simulink model "UAVModel"  (R2018a)
settings: Solver=ode45  StartTime=0.0  StopTime=400  RelTol=1e-3  EnableMultiTasking=on
libraries: simulink x3, dspsrcs4 x1
settings Model: Creator=leo  LastModifiedBy=e357599
settings DataIOCC: LimitDataPoints=on  SaveFormat=Array  SignalLoggingSaveFormat=ModelDataLogs
settings OptimizationCC: ExpressionDepthLimit=2147483647  LifeSpan=inf
settings DebuggingCC: UnderspecifiedInitializationDetection=Classic  MergeDetectMultiDrivingBlocksExec=none  SolverPrmCheckMsg=warning  FcnCallInpInsideContextMsg=warning  StateNameClashWarn=warning  SFUnexpectedBacktrackingDiag=warning  SFNoUnconditionalDefaultTransitionDiag=warning  SFExecutionAtInitializationDiag=none
settings HardwareCC: ProdBitPerPointer=32  ProdBitPerSizeT=32  ProdBitPerPtrDiffT=32  ProdLargestAtomicFloat=None  ProdIntDivRoundTo=Undefined  ProdEndianess=Unspecified  ProdWordSize=32  ProdHWDeviceType=32-bit Generic
settings ModelReferenceCC: PropagateSignalLabelsOutOfModel=off
settings CodeAppCC: StateflowObjectComments=on
settings GRTTargetCC: TargetLangStandard=C89/C90 (ANSI)  GeneratePreprocessorConditionals=Disable all  CombineOutputUpdateFcns=off  GRTInterface=on
settings ConfigComp: CovMetricSettings=dw  CovHtmlReporting=on  CovSaveCumulativeToWorkspaceVar=on  CovSaveSingleToWorkspaceVar=on  CovExternalEMLEnable=off

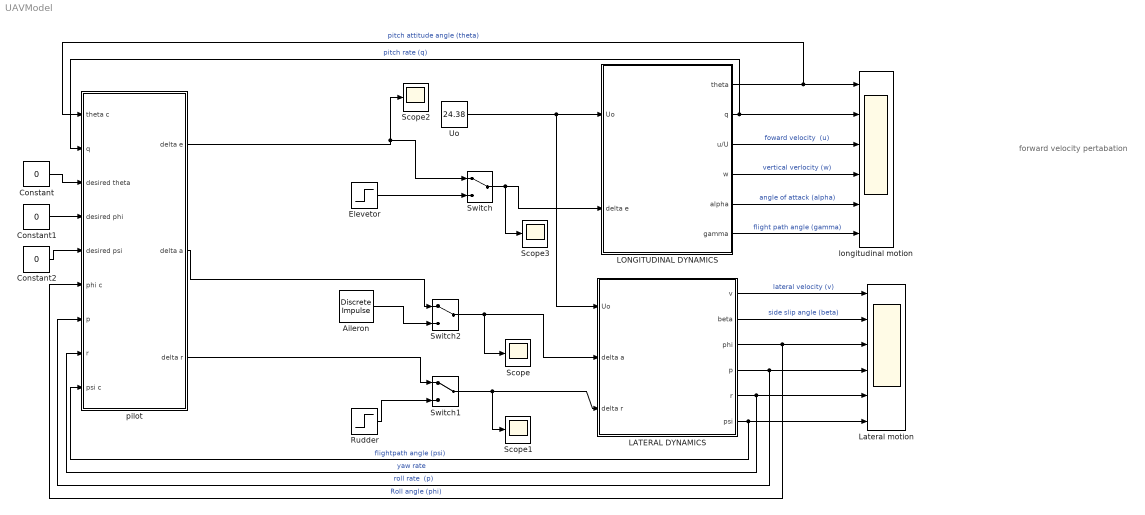
== system UAVModel ==
  note: forward velocity pertabation
  " Switch" : ManualSwitch
  " Switch1" : ManualSwitch
  " Switch2" : ManualSwitch
  Aileron : dspsrcs4/Discrete  Impulse  Delay=0  SampleTime=1  FrameSample=1  OutputFrames=off  dataType=double  isSigned=on  wordLen=16  udDataType=sfix(16)  fracBitsMode=Best precision  numFracBits=15  OutDataTypeStr=double  LastOutDataTypeStr=double
  Constant : Constant  Value=0  SampleTime=6
  Constant1 : Constant  Value=0
  Constant2 : Constant  Value=0
  Elevetor : Step  Time=0.5  After=-1  SampleTime=0
  LATERAL DYNAMICS : Subsystem
  LONGITUDINAL DYNAMICS : Subsystem
  Lateral motion : Scope  NumInputPorts=6
  Rudder : Step  Time=0.5  SampleTime=0
  Scope{,1..3} (4 alike) : Scope
  Uo : Constant  Value=24.38
  longitudinal motion : Scope  NumInputPorts=6
  "pilot " : Subsystem
  wires:
  " Switch"/1 -> Scope3/1, LONGITUDINAL DYNAMICS/2(delta e)
  Uo/1 -> LONGITUDINAL DYNAMICS/1(" Uo"), LATERAL DYNAMICS/1(Uo)
  Elevetor/1 -> " Switch"/2
  LONGITUDINAL DYNAMICS/6(gamma) -> longitudinal motion/6  "flight path angle (gamma)"
  " Switch1"/1 -> Scope1/1, LATERAL DYNAMICS/3(delta r)
  Rudder/1 -> " Switch1"/2
  LONGITUDINAL DYNAMICS/4(w) -> longitudinal motion/4  "vertical verlocity (w)"
  Constant1/1 -> "pilot "/4(desired phi)
  Constant2/1 -> "pilot "/5(desired psi)
  "pilot "/2(delta a) -> " Switch2"/1
  "pilot "/1(delta e) -> " Switch"/1, Scope2/1
  Constant/1 -> "pilot "/3(desired theta)
  "pilot "/3(delta r) -> " Switch1"/1
  LONGITUDINAL DYNAMICS/1(theta) -> longitudinal motion/1, "pilot "/1(theta c)  "pitch attitude angle (theta)"
  LONGITUDINAL DYNAMICS/2(q) -> longitudinal motion/2, "pilot "/2(q)  "pitch rate (q)"
  LONGITUDINAL DYNAMICS/3(u/U) -> longitudinal motion/3  "foward velocity  (u)"
  LONGITUDINAL DYNAMICS/5(alpha) -> longitudinal motion/5  "angle of attack (alpha)"
  LATERAL DYNAMICS/1(v) -> Lateral motion/1  "lateral velocity (v)"
  LATERAL DYNAMICS/2(beta) -> Lateral motion/2  "side slip angle (beta)"
  LATERAL DYNAMICS/3(phi) -> Lateral motion/3, "pilot "/6(phi c)  "Roll angle (phi)"
  LATERAL DYNAMICS/4(p) -> Lateral motion/4, "pilot "/7(p)  "roll rate  (p)"
  LATERAL DYNAMICS/5(r) -> Lateral motion/5, "pilot "/8(r)  "yaw rate"
  LATERAL DYNAMICS/6(psi) -> Lateral motion/6, "pilot "/9(psi c)  "flightpath angle (psi)"
  Aileron/1 -> " Switch2"/2
  " Switch2"/1 -> Scope/1, LATERAL DYNAMICS/2("delta a ")

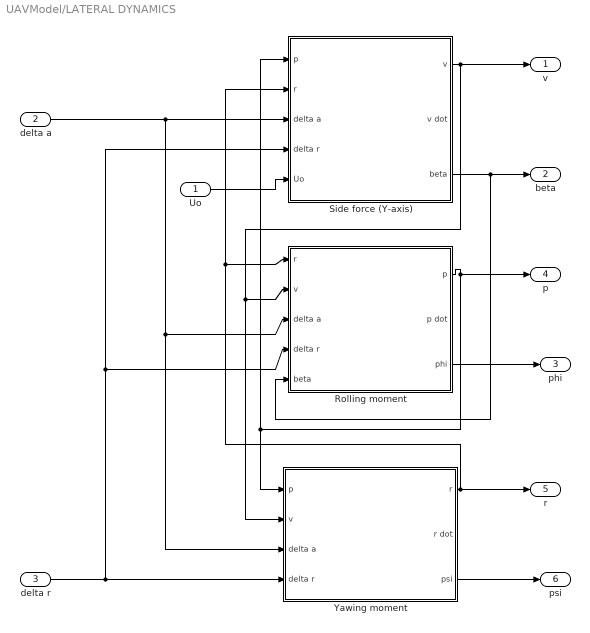
== system UAVModel/LATERAL DYNAMICS ==
  Uo : Inport
  "delta a " : Inport  Port=2
  delta r : Inport  Port=3
  Rolling moment : Subsystem
  Side force (Y-axis) : Subsystem
  Yawing moment : Subsystem
  v : Outport
  beta : Outport  Port=2
  phi : Outport  Port=3
  p : Outport  Port=4
  r : Outport  Port=5
  psi : Outport  Port=6
  wires:
  delta r/1 -> Side force (Y-axis)/4(delta r), Rolling moment/4(delta r), Yawing moment/4(delta r)
  "delta a "/1 -> Side force (Y-axis)/3(delta a), Rolling moment/3(delta a), Yawing moment/3(delta a)
  Uo/1 -> Side force (Y-axis)/5(Uo)
  Side force (Y-axis)/1(v) -> Rolling moment/2(v), Yawing moment/2(v), v/1
  Rolling moment/1(p) -> Yawing moment/1(p), Side force (Y-axis)/1(p), p/1
  Yawing moment/1(r) -> Rolling moment/1(r), Side force (Y-axis)/2(r), r/1
  Side force (Y-axis)/3(beta) -> beta/1, Rolling moment/5(beta)
  Yawing moment/3(psi) -> psi/1
  Rolling moment/3(phi) -> phi/1

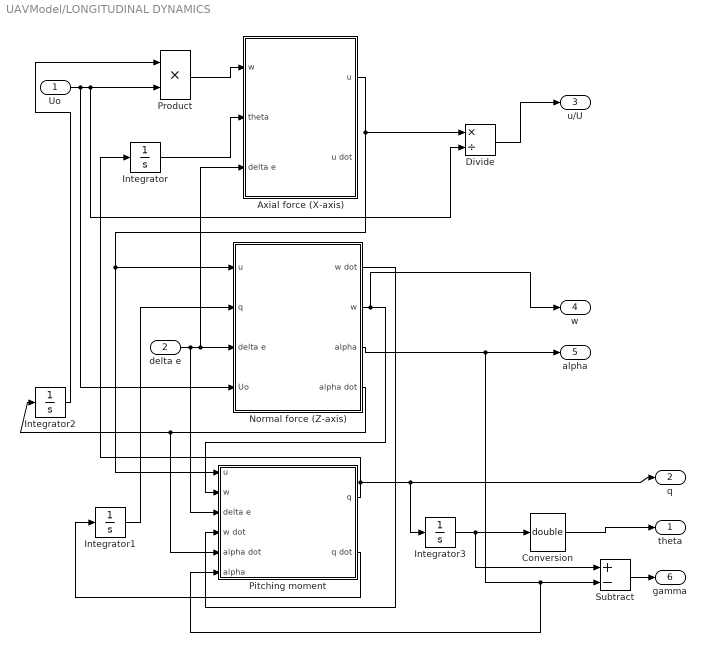
== system UAVModel/LONGITUDINAL DYNAMICS ==
  " Uo" : Inport
  delta e : Inport  Port=2
  " Conversion" : DataTypeConversion  OutDataTypeStr=double
  Axial force (X-axis) : Subsystem
  Divide : Product  Inputs=*/
  Integrator{,1..3} (4 alike) : Integrator
  "Normal force (Z-axis) " : Subsystem
  Pitching moment : Subsystem
  Product : Product  RndMeth=Zero
  Subtract : Sum  Inputs=+-
  theta : Outport
  q : Outport  Port=2
  u/U : Outport  Port=3
  w : Outport  Port=4
  alpha : Outport  Port=5
  gamma : Outport  Port=6
  wires:
  " Uo"/1 -> "Normal force (Z-axis) "/4(Uo), Product/2, Divide/2
  delta e/1 -> Pitching moment/3(delta e), "Normal force (Z-axis) "/3(delta e), Axial force (X-axis)/3(delta e)
  Product/1 -> Axial force (X-axis)/1(w)
  Axial force (X-axis)/1(u) -> Pitching moment/1(u), "Normal force (Z-axis) "/1(u), Divide/1
  "Normal force (Z-axis) "/2(w) -> Pitching moment/2(w), w/1
  "Normal force (Z-axis) "/1(w dot) -> Pitching moment/4(w dot)
  Pitching moment/1(q) -> Integrator/1, q/1, Integrator3/1
  Integrator/1 -> Axial force (X-axis)/2(theta)
  Integrator1/1 -> "Normal force (Z-axis) "/2(q)
  Pitching moment/2(q dot) -> Integrator1/1
  "Normal force (Z-axis) "/3(alpha) -> alpha/1, Subtract/2, Pitching moment/6("alpha ")
  Integrator2/1 -> Product/1
  "Normal force (Z-axis) "/4(alpha dot) -> Integrator2/1, Pitching moment/5(alpha dot)
  Integrator3/1 -> Subtract/1, " Conversion"/1
  Subtract/1 -> gamma/1
  " Conversion"/1 -> theta/1
  Divide/1 -> u/U/1

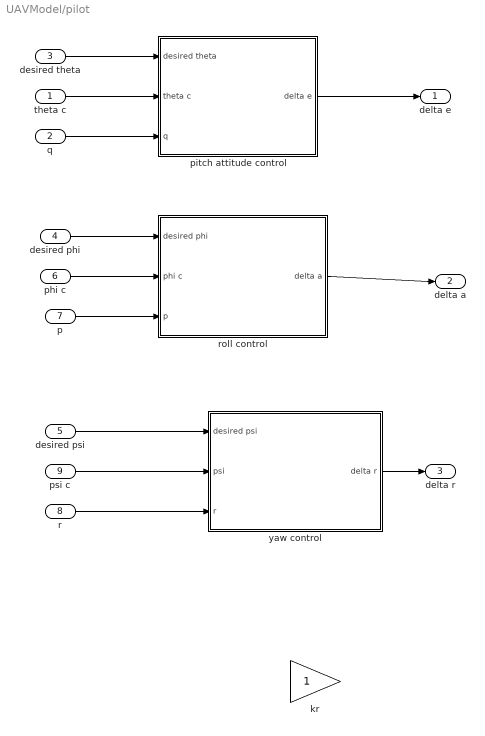
== system UAVModel/pilot  ==
  theta c : Inport
  q : Inport  Port=2
  desired theta : Inport  Port=3
  desired phi : Inport  Port=4
  desired psi : Inport  Port=5
  phi c : Inport  Port=6
  p : Inport  Port=7
  r : Inport  Port=8
  psi c : Inport  Port=9
  kr : Gain
  pitch attitude control : Subsystem
  roll control : Subsystem
  yaw control : Subsystem
  delta e : Outport
  delta a : Outport  Port=2
  delta r : Outport  Port=3
  wires:
  desired theta/1 -> pitch attitude control/1(desired theta)
  theta c/1 -> pitch attitude control/2(theta c)
  q/1 -> pitch attitude control/3(q)
  desired phi/1 -> roll control/1("desired phi ")
  phi c/1 -> roll control/2(phi c)
  p/1 -> roll control/3(p)
  desired psi/1 -> yaw control/1("desired psi ")
  psi c/1 -> yaw control/2(psi)
  r/1 -> yaw control/3(r)
  roll control/1(delta a) -> delta a/1
  pitch attitude control/1(delta e) -> delta e/1
  yaw control/1(delta r) -> delta r/1

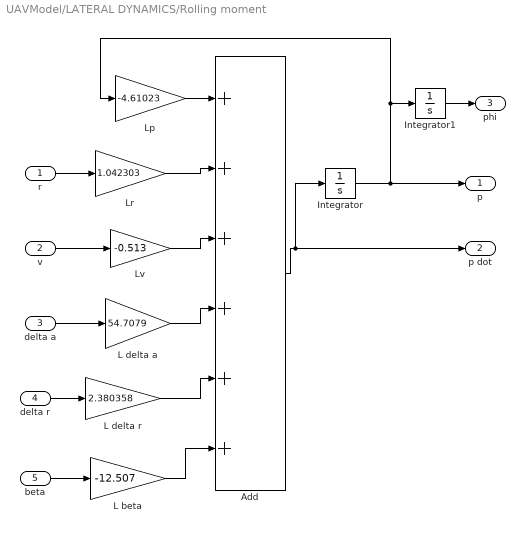
== system UAVModel/LATERAL DYNAMICS/Rolling moment ==
  r : Inport
  v : Inport  Port=2
  delta a : Inport  Port=3
  delta r : Inport  Port=4
  beta : Inport  Port=5
  Add : Sum  Inputs=++++++
  Integrator : Integrator
  Integrator1 : Integrator
  L beta : Gain  Gain=-12.507
  "L delta a " : Gain  Gain=54.7079
  L delta r : Gain  Gain=2.380358
  Lp : Gain  Gain=-4.61023
  Lr : Gain  Gain=1.042303
  Lv : Gain  Gain=-0.513
  p : Outport
  p dot : Outport  Port=2
  phi : Outport  Port=3
  wires:
  Add/1 -> p dot/1, Integrator/1
  Lp/1 -> Add/1
  Lr/1 -> Add/2
  Lv/1 -> Add/3
  "L delta a "/1 -> Add/4
  L delta r/1 -> Add/5
  delta r/1 -> L delta r/1
  delta a/1 -> "L delta a "/1
  v/1 -> Lv/1
  r/1 -> Lr/1
  Integrator/1 -> p/1, Lp/1, Integrator1/1
  Integrator1/1 -> phi/1
  L beta/1 -> Add/6
  beta/1 -> L beta/1

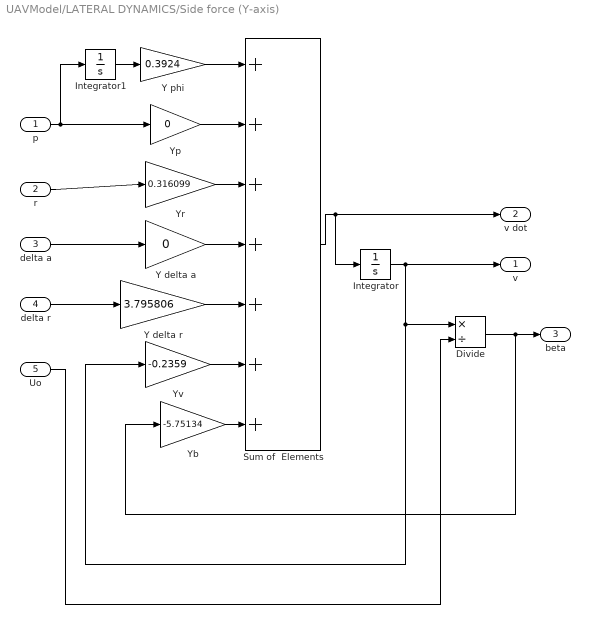
== system UAVModel/LATERAL DYNAMICS/Side force (Y-axis) ==
  p : Inport
  r : Inport  Port=2
  delta a : Inport  Port=3
  delta r : Inport  Port=4
  Uo : Inport  Port=5
  Divide : Product  Inputs=*/
  Integrator : Integrator
  Integrator1 : Integrator
  Sum of  Elements : Sum  Inputs=+++++++
  Y delta a : Gain  Gain=0
  Y delta r : Gain  Gain=3.795806
  Y phi : Gain  Gain=0.3924
  Yb : Gain  Gain=-5.75134
  Yp : Gain  Gain=0
  Yr : Gain  Gain=0.316099
  Yv : Gain  Gain=-0.2359
  v : Outport
  v dot : Outport  Port=2
  beta : Outport  Port=3
  wires:
  Sum of  Elements/1 -> v dot/1, Integrator/1
  Integrator/1 -> v/1, Divide/1, Yv/1
  Yv/1 -> Sum of  Elements/6
  Y delta r/1 -> Sum of  Elements/5
  Y delta a/1 -> Sum of  Elements/4
  Yr/1 -> Sum of  Elements/3
  Yp/1 -> Sum of  Elements/2
  Y phi/1 -> Sum of  Elements/1
  r/1 -> Yr/1
  p/1 -> Yp/1, Integrator1/1
  Integrator1/1 -> Y phi/1
  delta a/1 -> Y delta a/1
  delta r/1 -> Y delta r/1
  Uo/1 -> Divide/2
  Divide/1 -> beta/1, Yb/1
  Yb/1 -> Sum of  Elements/7

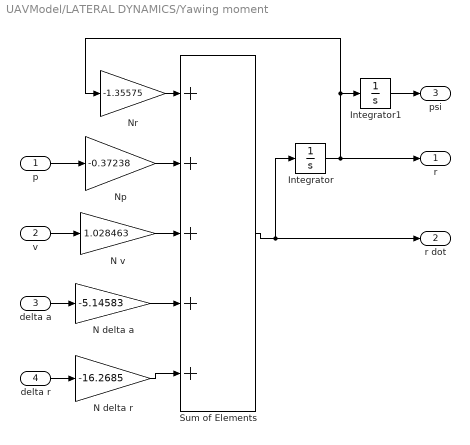
== system UAVModel/LATERAL DYNAMICS/Yawing moment ==
  p : Inport
  v : Inport  Port=2
  delta a : Inport  Port=3
  delta r : Inport  Port=4
  Integrator : Integrator
  Integrator1 : Integrator
  N delta a : Gain  Gain=-5.14583
  N delta r : Gain  Gain=-16.2685
  N v : Gain  Gain=1.028463
  Np : Gain  Gain=-0.37238
  Nr : Gain  Gain=-1.35575
  Sum of Elements : Sum  Inputs=+++++
  r : Outport
  r dot : Outport  Port=2
  psi : Outport  Port=3
  wires:
  Sum of Elements/1 -> Integrator/1, r dot/1
  Integrator/1 -> r/1, Nr/1, Integrator1/1
  delta r/1 -> N delta r/1
  delta a/1 -> N delta a/1
  v/1 -> N v/1
  p/1 -> Np/1
  Nr/1 -> Sum of Elements/1
  Np/1 -> Sum of Elements/2
  N v/1 -> Sum of Elements/3
  N delta a/1 -> Sum of Elements/4
  N delta r/1 -> Sum of Elements/5
  Integrator1/1 -> psi/1

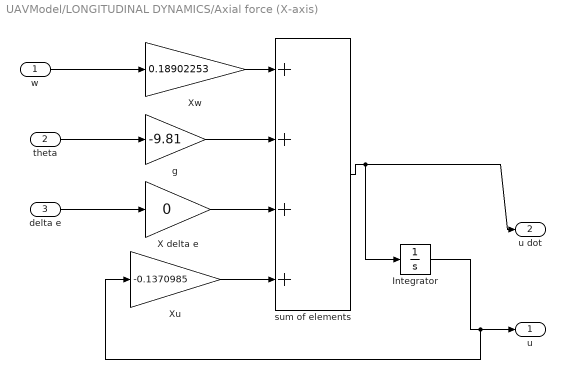
== system UAVModel/LONGITUDINAL DYNAMICS/Axial force (X-axis) ==
  w : Inport
  theta : Inport  Port=2
  delta e : Inport  Port=3
  Integrator : Integrator
  X delta e : Gain  Gain=0
  Xu : Gain  RequirementInfo={} %GIDa_afb63dbf_c4f0_45b2_8257_9555063e987b  Gain=-0.1370985
  Xw : Gain  Gain=0.18902253
  g : Gain  Gain=-9.81
  sum of elements : Sum  Inputs=++++
  u : Outport
  u dot : Outport  Port=2
  wires:
  Xw/1 -> sum of elements/1
  w/1 -> Xw/1
  g/1 -> sum of elements/2
  sum of elements/1 -> Integrator/1, u dot/1
  Integrator/1 -> Xu/1, u/1
  theta/1 -> g/1
  Xu/1 -> sum of elements/4
  X delta e/1 -> sum of elements/3
  delta e/1 -> X delta e/1

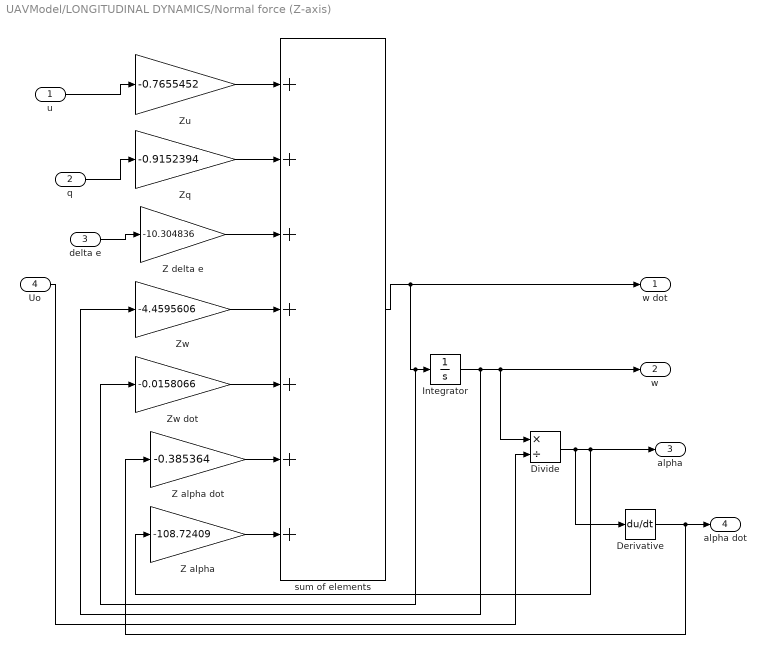
== system UAVModel/LONGITUDINAL DYNAMICS/Normal force (Z-axis)  ==
  u : Inport
  q : Inport  Port=2
  delta e : Inport  Port=3
  Uo : Inport  Port=4
  Derivative : Derivative
  Divide : Product  Inputs=*/
  Integrator : Integrator
  Z alpha : Gain  Gain=-108.72409
  Z alpha dot : Gain  Gain=-0.385364
  Z delta e : Gain  Gain=-10.304836
  Zq : Gain  Gain=-0.9152394
  Zu : Gain  Gain=-0.7655452
  Zw : Gain  Gain=-4.4595606
  Zw dot : Gain  Gain=-0.0158066
  sum of elements : Sum  Inputs=+++++++
  w dot : Outport
  w : Outport  Port=2
  alpha : Outport  Port=3
  alpha dot : Outport  Port=4
  wires:
  Zu/1 -> sum of elements/1
  u/1 -> Zu/1
  Zq/1 -> sum of elements/2
  q/1 -> Zq/1
  Z delta e/1 -> sum of elements/3
  delta e/1 -> Z delta e/1
  Zw/1 -> sum of elements/4
  sum of elements/1 -> w dot/1, Integrator/1, Zw dot/1
  Integrator/1 -> w/1, Divide/1, Zw/1
  Uo/1 -> Divide/2
  Divide/1 -> Derivative/1, alpha/1, Z alpha/1
  Derivative/1 -> alpha dot/1, Z alpha dot/1
  Zw dot/1 -> sum of elements/5
  Z alpha dot/1 -> sum of elements/6
  Z alpha/1 -> sum of elements/7

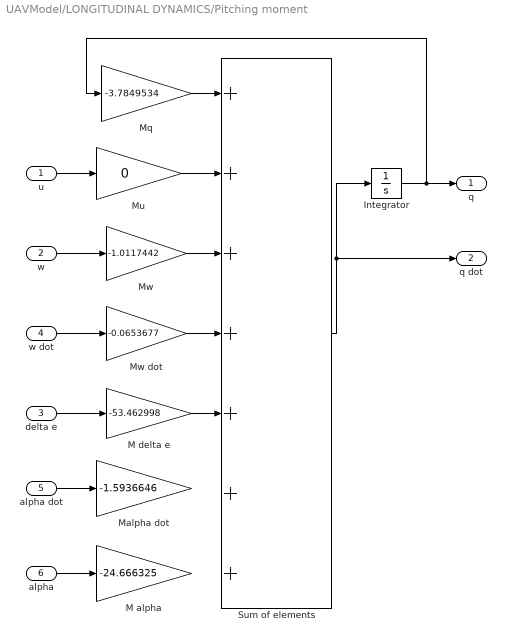
== system UAVModel/LONGITUDINAL DYNAMICS/Pitching moment ==
  u : Inport
  w : Inport  Port=2
  delta e : Inport  Port=3
  w dot : Inport  Port=4
  alpha dot : Inport  Port=5
  "alpha " : Inport  Port=6
  Integrator : Integrator
  M alpha : Gain  Gain=-24.666325
  M delta e : Gain  Gain=-53.462998
  Malpha dot : Gain  Gain=-1.5936646
  Mq : Gain  Gain=-3.7849534
  Mu : Gain  Gain=0
  Mw : Gain  Gain=-1.0117442
  Mw dot : Gain  Gain=-0.0653677
  "Sum of elements " : Sum  Inputs=+++++++
  q : Outport
  q dot : Outport  Port=2
  wires:
  w/1 -> Mw/1
  u/1 -> Mu/1
  w dot/1 -> Mw dot/1
  delta e/1 -> M delta e/1
  M delta e/1 -> "Sum of elements "/5
  Mw dot/1 -> "Sum of elements "/4
  Mw/1 -> "Sum of elements "/3
  Mu/1 -> "Sum of elements "/2
  Mq/1 -> "Sum of elements "/1
  "Sum of elements "/1 -> q dot/1, Integrator/1
  Integrator/1 -> q/1, Mq/1
  alpha dot/1 -> Malpha dot/1
  "alpha "/1 -> M alpha/1

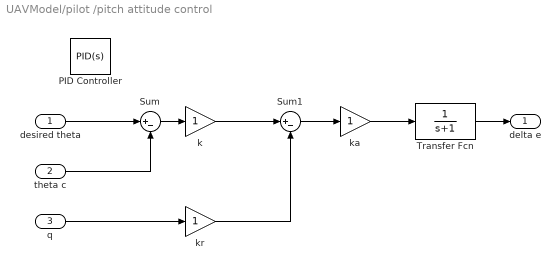
== system UAVModel/pilot /pitch attitude control ==
  desired theta : Inport
  theta c : Inport  Port=2
  q : Inport  Port=3
  PID Controller : simulink/Continuous/PID Controller  Controller=PID  TimeDomain=Continuous-time  SampleTime=-1  IntegratorMethod=Forward Euler  FilterMethod=Forward Euler  Form=Parallel  UseFilter=on  ControllerParametersSource=internal  P=1  I=1  D=0  N=100  InitialConditionSource=internal  InitialConditionForIntegrator=0  InitialConditionForFilter=0  ExternalReset=none  LimitOutput=off  UpperSaturationLimit=inf  LowerSaturationLimit=-inf  LinearizeAsGain=off  AntiWindupMode=none  Kb=1  TrackingMode=off  Kt=1  PParamMin=[]  PParamMax=[]  IParamMin=[]  IParamMax=[]  DParamMin=[]  DParamMax=[]  NParamMin=[]  NParamMax=[]  KbParamMin=[]  KbParamMax=[]  KtParamMin=[]  KtParamMax=[]  POutMin=[]  POutMax=[]  IOutMin=[]  IOutMax=[]  DOutMin=[]  DOutMax=[]  NOutMin=[]  NOutMax=[]  KbOutMin=[]  KbOutMax=[]  KtOutMin=[]  KtOutMax=[]  IntegratorOutMin=[]  IntegratorOutMax=[]  FilterOutMin=[]  FilterOutMax=[]  SumOutMin=[]  SumOutMax=[]  SumI1OutMin=[]  SumI1OutMax=[]  SumI2OutMin=[]  SumI2OutMax=[]  SumI3OutMin=[]  SumI3OutMax=[]  SumDOutMin=[]  SumDOutMax=[]  SaturationOutMin=[]  SaturationOutMax=[]  IntegratorContinuousStateAttributes=''  IntegratorStateMustResolveToSignalObject=off  IntegratorRTWStateStorageClass=Auto  FilterContinuousStateAttributes=''  FilterStateMustResolveToSignalObject=off  FilterRTWStateStorageClass=Auto  DifferentiatorICPrevScaledInput=0  DifferentiatorOutMin=[]  DifferentiatorOutMax=[]  FilterDiffOutCoefMin=[]  FilterDiffOutCoefMax=[]  SumDenOutMin=[]  SumDenOutMax=[]  SumNumOutMin=[]  SumNumOutMax=[]  ReciprocalOutMin=[]  ReciprocalOutMax=[]  DivideOutMin=[]  DivideOutMax=[]  TunerSelectOption=Transfer Function Based (PID Tuner App)
  Sum : Sum  Inputs=|+-
  Sum1 : Sum  Inputs=|+-
  Transfer Fcn : TransferFcn  Denominator=[1 1]
  k : Gain
  ka : Gain
  kr : Gain
  delta e : Outport
  wires:
  Transfer Fcn/1 -> delta e/1
  ka/1 -> Transfer Fcn/1
  Sum1/1 -> ka/1
  desired theta/1 -> Sum/1
  kr/1 -> Sum1/2
  theta c/1 -> Sum/2
  q/1 -> kr/1
  Sum/1 -> k/1
  k/1 -> Sum1/1

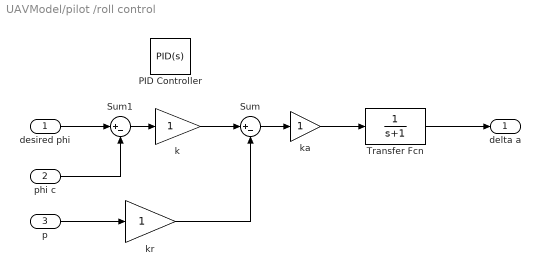
== system UAVModel/pilot /roll control ==
  "desired phi " : Inport
  phi c : Inport  Port=2
  p : Inport  Port=3
  PID Controller : simulink/Continuous/PID Controller  Controller=PID  TimeDomain=Continuous-time  SampleTime=-1  IntegratorMethod=Forward Euler  FilterMethod=Forward Euler  Form=Parallel  UseFilter=on  ControllerParametersSource=internal  P=1  I=1  D=0  N=100  InitialConditionSource=internal  InitialConditionForIntegrator=0  InitialConditionForFilter=0  ExternalReset=none  LimitOutput=off  UpperSaturationLimit=inf  LowerSaturationLimit=-inf  LinearizeAsGain=off  AntiWindupMode=none  Kb=1  TrackingMode=off  Kt=1  PParamMin=[]  PParamMax=[]  IParamMin=[]  IParamMax=[]  DParamMin=[]  DParamMax=[]  NParamMin=[]  NParamMax=[]  KbParamMin=[]  KbParamMax=[]  KtParamMin=[]  KtParamMax=[]  POutMin=[]  POutMax=[]  IOutMin=[]  IOutMax=[]  DOutMin=[]  DOutMax=[]  NOutMin=[]  NOutMax=[]  KbOutMin=[]  KbOutMax=[]  KtOutMin=[]  KtOutMax=[]  IntegratorOutMin=[]  IntegratorOutMax=[]  FilterOutMin=[]  FilterOutMax=[]  SumOutMin=[]  SumOutMax=[]  SumI1OutMin=[]  SumI1OutMax=[]  SumI2OutMin=[]  SumI2OutMax=[]  SumI3OutMin=[]  SumI3OutMax=[]  SumDOutMin=[]  SumDOutMax=[]  SaturationOutMin=[]  SaturationOutMax=[]  IntegratorContinuousStateAttributes=''  IntegratorStateMustResolveToSignalObject=off  IntegratorRTWStateStorageClass=Auto  FilterContinuousStateAttributes=''  FilterStateMustResolveToSignalObject=off  FilterRTWStateStorageClass=Auto  DifferentiatorICPrevScaledInput=0  DifferentiatorOutMin=[]  DifferentiatorOutMax=[]  FilterDiffOutCoefMin=[]  FilterDiffOutCoefMax=[]  SumDenOutMin=[]  SumDenOutMax=[]  SumNumOutMin=[]  SumNumOutMax=[]  ReciprocalOutMin=[]  ReciprocalOutMax=[]  DivideOutMin=[]  DivideOutMax=[]  TunerSelectOption=Transfer Function Based (PID Tuner App)
  Sum : Sum  Inputs=|+-
  Sum1 : Sum  Inputs=|+-
  Transfer Fcn : TransferFcn  Denominator=[1 1]
  k : Gain
  ka : Gain
  kr : Gain
  delta a : Outport
  wires:
  ka/1 -> Transfer Fcn/1
  Transfer Fcn/1 -> delta a/1
  Sum/1 -> ka/1
  "desired phi "/1 -> Sum1/1
  p/1 -> kr/1
  kr/1 -> Sum/2
  phi c/1 -> Sum1/2
  k/1 -> Sum/1
  Sum1/1 -> k/1

== system UAVModel/pilot /yaw control ==
  "desired psi " : Inport
  psi : Inport  Port=2
  r : Inport  Port=3
  KR : Gain
  Ka : Gain
  PID Controller : simulink/Continuous/PID Controller  Controller=PID  TimeDomain=Continuous-time  SampleTime=-1  IntegratorMethod=Forward Euler  FilterMethod=Forward Euler  Form=Parallel  UseFilter=on  ControllerParametersSource=internal  P=1  I=1  D=0  N=100  InitialConditionSource=internal  InitialConditionForIntegrator=0  InitialConditionForFilter=0  ExternalReset=none  LimitOutput=off  UpperSaturationLimit=inf  LowerSaturationLimit=-inf  LinearizeAsGain=off  AntiWindupMode=none  Kb=1  TrackingMode=off  Kt=1  PParamMin=[]  PParamMax=[]  IParamMin=[]  IParamMax=[]  DParamMin=[]  DParamMax=[]  NParamMin=[]  NParamMax=[]  KbParamMin=[]  KbParamMax=[]  KtParamMin=[]  KtParamMax=[]  POutMin=[]  POutMax=[]  IOutMin=[]  IOutMax=[]  DOutMin=[]  DOutMax=[]  NOutMin=[]  NOutMax=[]  KbOutMin=[]  KbOutMax=[]  KtOutMin=[]  KtOutMax=[]  IntegratorOutMin=[]  IntegratorOutMax=[]  FilterOutMin=[]  FilterOutMax=[]  SumOutMin=[]  SumOutMax=[]  SumI1OutMin=[]  SumI1OutMax=[]  SumI2OutMin=[]  SumI2OutMax=[]  SumI3OutMin=[]  SumI3OutMax=[]  SumDOutMin=[]  SumDOutMax=[]  SaturationOutMin=[]  SaturationOutMax=[]  IntegratorContinuousStateAttributes=''  IntegratorStateMustResolveToSignalObject=off  IntegratorRTWStateStorageClass=Auto  FilterContinuousStateAttributes=''  FilterStateMustResolveToSignalObject=off  FilterRTWStateStorageClass=Auto  DifferentiatorICPrevScaledInput=0  DifferentiatorOutMin=[]  DifferentiatorOutMax=[]  FilterDiffOutCoefMin=[]  FilterDiffOutCoefMax=[]  SumDenOutMin=[]  SumDenOutMax=[]  SumNumOutMin=[]  SumNumOutMax=[]  ReciprocalOutMin=[]  ReciprocalOutMax=[]  DivideOutMin=[]  DivideOutMax=[]  TunerSelectOption=Transfer Function Based (PID Tuner App)
  Sum : Sum  Inputs=|+-
  Sum1 : Sum  Inputs=|+-
  Transfer Fcn : TransferFcn  Denominator=[1 1]
  kr : Gain
  delta r : Outport
  wires:
  "desired psi "/1 -> Sum/1
  Sum1/1 -> Ka/1
  Ka/1 -> Transfer Fcn/1
  Transfer Fcn/1 -> delta r/1
  r/1 -> KR/1
  KR/1 -> Sum1/2
  psi/1 -> Sum/2
  kr/1 -> Sum1/1
  Sum/1 -> kr/1
